simulink model "TestCase_TestSpace_TestSpace_mapping"  (R2016b)
settings: Solver=FixedStepAuto  StartTime=0.0  StopTime=10.0  RelTol=1e-3
model workspace: external: MAT-File TestCase_TestSpace_TestSpace_mapping.mat (data not in the file)
libraries: libTLAsserts x4, libAsserts x2
settings Model: Creator=NEATdemo  LastModifiedBy=NEATdemo

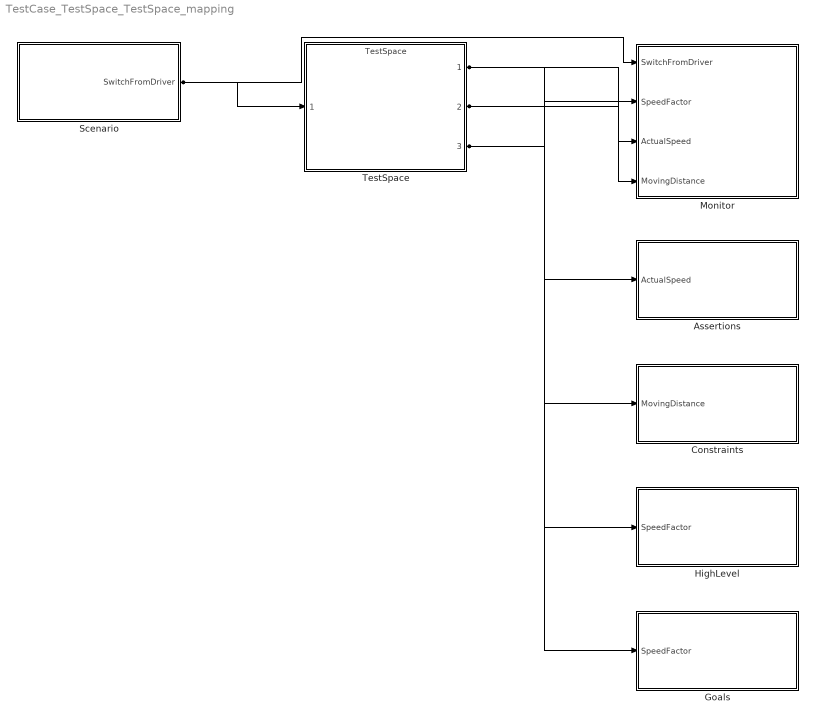
== system TestCase_TestSpace_TestSpace_mapping ==
  Assertions : Subsystem
  Constraints : Subsystem
  Goals : Subsystem
  HighLevel : Subsystem
  Monitor : Subsystem
  Scenario : Subsystem
  TestSpace : ModelReference  ModelNameDialog=TestSpace  SimulationMode=Normal  ModelReferenceVersion=1.13
  wires:
  Scenario/1(SwitchFromDriver) -> TestSpace/1, Monitor/1(SwitchFromDriver)
  TestSpace/3 -> Monitor/2(SpeedFactor), HighLevel/1(SpeedFactor), Goals/1(SpeedFactor)
  TestSpace/2 -> Monitor/3(ActualSpeed), Assertions/1(ActualSpeed)
  TestSpace/1 -> Monitor/4(MovingDistance), Constraints/1(MovingDistance)

== system TestCase_TestSpace_TestSpace_mapping/Assertions ==
  ActualSpeed : Inport
  assert_1 : Subsystem
  simout_1 : ToFile  Filename=assert_1.mat  MatrixName=assert_1  SaveFormat=Timeseries
  wires:
  ActualSpeed/1 -> assert_1/1(ActualSpeed)
  assert_1/1(assert_1_FAILED) -> simout_1/1

== system TestCase_TestSpace_TestSpace_mapping/Constraints ==
  MovingDistance : Inport
  const_1 : Subsystem
  simout_1 : ToFile  Filename=const_1.mat  MatrixName=const_1  SaveFormat=Timeseries
  wires:
  MovingDistance/1 -> const_1/1(MovingDistance)
  const_1/1(const_1_FAILED) -> simout_1/1

== system TestCase_TestSpace_TestSpace_mapping/Goals ==
  SpeedFactor : Inport
  goals_1 : Subsystem
  simout_1 : ToFile  Filename=goals_1.mat  MatrixName=goals_1  SaveFormat=Timeseries
  wires:
  SpeedFactor/1 -> goals_1/1(SpeedFactor)
  goals_1/1(goals_1_VAL) -> simout_1/1

== system TestCase_TestSpace_TestSpace_mapping/HighLevel ==
  SpeedFactor : Inport
  highlevel_1 : Subsystem
  simout_1 : ToFile  Filename=highlevel_1.mat  MatrixName=highlevel_1  SaveFormat=Timeseries
  wires:
  SpeedFactor/1 -> highlevel_1/1(SpeedFactor)
  highlevel_1/1(highlevel_1_FAILED) -> simout_1/1

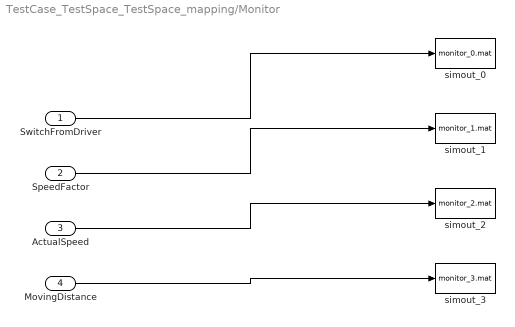
== system TestCase_TestSpace_TestSpace_mapping/Monitor ==
  SwitchFromDriver : Inport
  SpeedFactor : Inport  Port=2
  ActualSpeed : Inport  Port=3
  MovingDistance : Inport  Port=4
  simout_0 : ToFile  Filename=monitor_0.mat  MatrixName=SwitchFromDriver  SaveFormat=Timeseries
  simout_1 : ToFile  Filename=monitor_1.mat  MatrixName=SpeedFactor  SaveFormat=Timeseries
  simout_2 : ToFile  Filename=monitor_2.mat  MatrixName=ActualSpeed  SaveFormat=Timeseries
  simout_3 : ToFile  Filename=monitor_3.mat  MatrixName=MovingDistance  SaveFormat=Timeseries
  wires:
  SwitchFromDriver/1 -> simout_0/1
  SpeedFactor/1 -> simout_1/1
  ActualSpeed/1 -> simout_2/1
  MovingDistance/1 -> simout_3/1

== system TestCase_TestSpace_TestSpace_mapping/Scenario ==
  Scenario : Stateflow chart  TreatAsAtomicUnit=on
  clock : Clock
  SwitchFromDriver : Outport
  wires:
  Scenario/1(SwitchFromDriver) -> SwitchFromDriver/1
  clock/1 -> Scenario/1(clk)

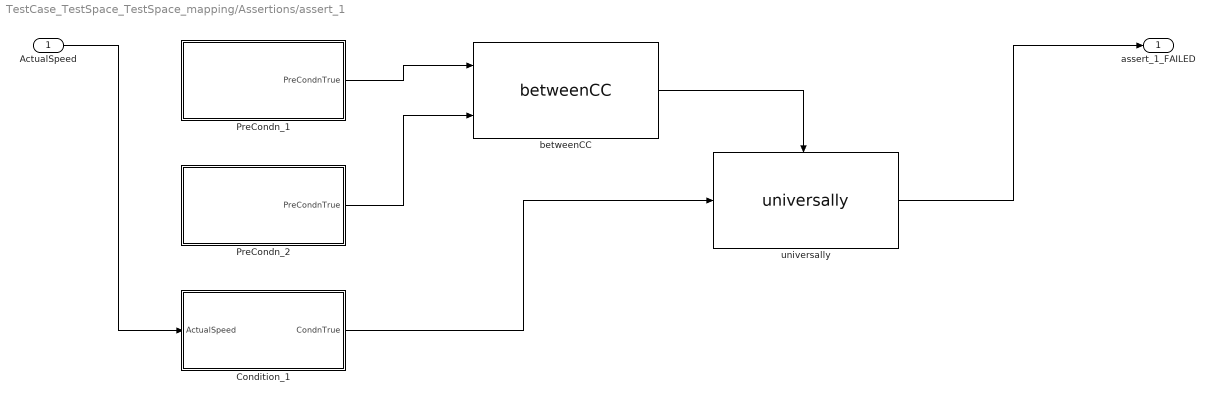
== system TestCase_TestSpace_TestSpace_mapping/Assertions/assert_1 ==
  ActualSpeed : Inport
  Condition_1 : Subsystem
  PreCondn_1 : Subsystem
  PreCondn_2 : Subsystem
  betweenCC : libTLAsserts/betweenCC
  universally : libTLAsserts/universally
  assert_1_FAILED : Outport
  wires:
  ActualSpeed/1 -> Condition_1/1(ActualSpeed)
  PreCondn_1/1(PreCondnTrue) -> betweenCC/1
  PreCondn_2/1(PreCondnTrue) -> betweenCC/2
  Condition_1/1(CondnTrue) -> universally/1
  betweenCC/1 -> universally/Enable
  universally/1 -> assert_1_FAILED/1

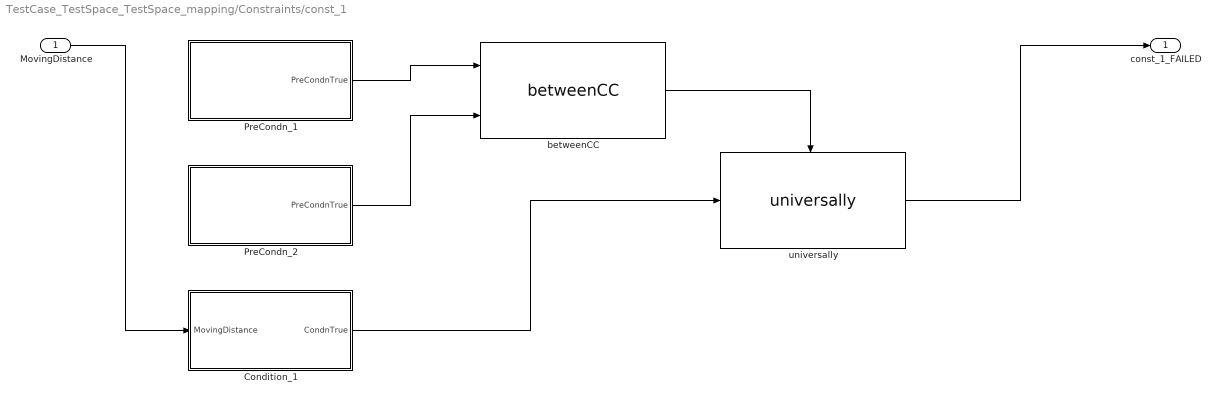
== system TestCase_TestSpace_TestSpace_mapping/Constraints/const_1 ==
  MovingDistance : Inport
  Condition_1 : Subsystem
  PreCondn_1 : Subsystem
  PreCondn_2 : Subsystem
  betweenCC : libTLAsserts/betweenCC
  universally : libTLAsserts/universally
  const_1_FAILED : Outport
  wires:
  MovingDistance/1 -> Condition_1/1(MovingDistance)
  PreCondn_1/1(PreCondnTrue) -> betweenCC/1
  PreCondn_2/1(PreCondnTrue) -> betweenCC/2
  Condition_1/1(CondnTrue) -> universally/1
  betweenCC/1 -> universally/Enable
  universally/1 -> const_1_FAILED/1

== system TestCase_TestSpace_TestSpace_mapping/Goals/goals_1 ==
  SpeedFactor : Inport
  goals_1_VAL : Outport
  wires:
  SpeedFactor/1 -> goals_1_VAL/1

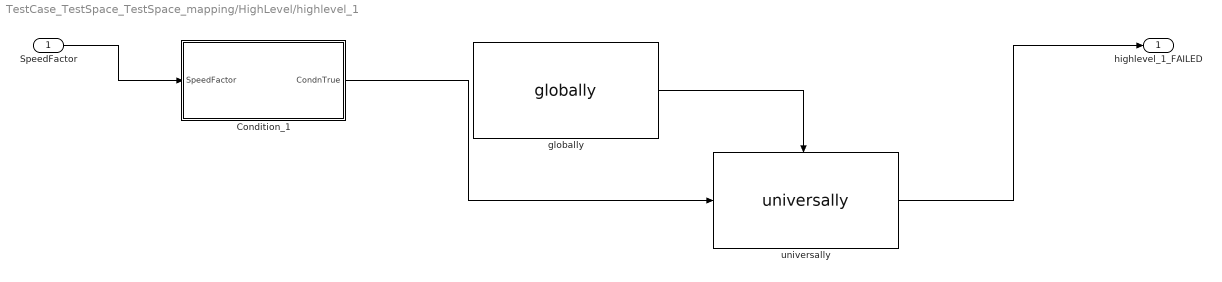
== system TestCase_TestSpace_TestSpace_mapping/HighLevel/highlevel_1 ==
  SpeedFactor : Inport
  Condition_1 : Subsystem
  globally : libAsserts/globally
  universally : libAsserts/universally
  highlevel_1_FAILED : Outport
  wires:
  SpeedFactor/1 -> Condition_1/1(SpeedFactor)
  Condition_1/1(CondnTrue) -> universally/1
  universally/1 -> highlevel_1_FAILED/1
  globally/1 -> universally/Enable

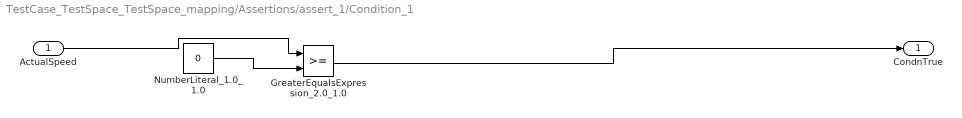
== system TestCase_TestSpace_TestSpace_mapping/Assertions/assert_1/Condition_1 ==
  ActualSpeed : Inport
  GreaterEqualsExpression_2.0_1.0 : RelationalOperator  OutDataTypeStr=boolean  RndMeth=Simplest
  NumberLiteral_1.0_1.0 : Constant  Value=0
  CondnTrue : Outport
  wires:
  ActualSpeed/1 -> GreaterEqualsExpression_2.0_1.0/1
  NumberLiteral_1.0_1.0/1 -> GreaterEqualsExpression_2.0_1.0/2
  GreaterEqualsExpression_2.0_1.0/1 -> CondnTrue/1

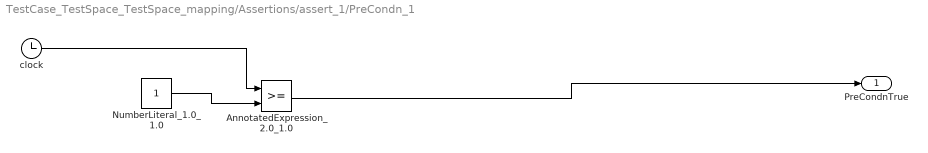
== system TestCase_TestSpace_TestSpace_mapping/Assertions/assert_1/PreCondn_1 ==
  AnnotatedExpression_2.0_1.0 : RelationalOperator  OutDataTypeStr=boolean  RndMeth=Simplest
  NumberLiteral_1.0_1.0 : Constant
  clock : Clock
  PreCondnTrue : Outport
  wires:
  clock/1 -> AnnotatedExpression_2.0_1.0/1
  NumberLiteral_1.0_1.0/1 -> AnnotatedExpression_2.0_1.0/2
  AnnotatedExpression_2.0_1.0/1 -> PreCondnTrue/1

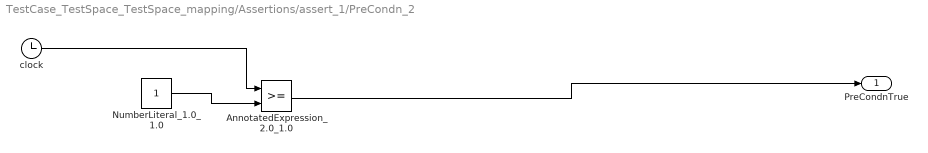
== system TestCase_TestSpace_TestSpace_mapping/Assertions/assert_1/PreCondn_2 ==
  AnnotatedExpression_2.0_1.0 : RelationalOperator  OutDataTypeStr=boolean  RndMeth=Simplest
  NumberLiteral_1.0_1.0 : Constant
  clock : Clock
  PreCondnTrue : Outport
  wires:
  clock/1 -> AnnotatedExpression_2.0_1.0/1
  NumberLiteral_1.0_1.0/1 -> AnnotatedExpression_2.0_1.0/2
  AnnotatedExpression_2.0_1.0/1 -> PreCondnTrue/1

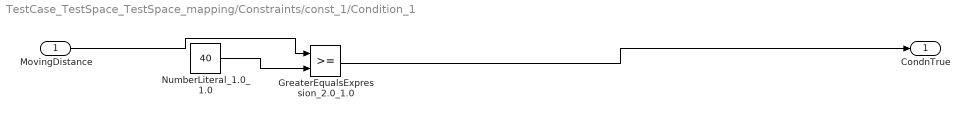
== system TestCase_TestSpace_TestSpace_mapping/Constraints/const_1/Condition_1 ==
  MovingDistance : Inport
  GreaterEqualsExpression_2.0_1.0 : RelationalOperator  OutDataTypeStr=boolean  RndMeth=Simplest
  NumberLiteral_1.0_1.0 : Constant  Value=40
  CondnTrue : Outport
  wires:
  MovingDistance/1 -> GreaterEqualsExpression_2.0_1.0/1
  NumberLiteral_1.0_1.0/1 -> GreaterEqualsExpression_2.0_1.0/2
  GreaterEqualsExpression_2.0_1.0/1 -> CondnTrue/1

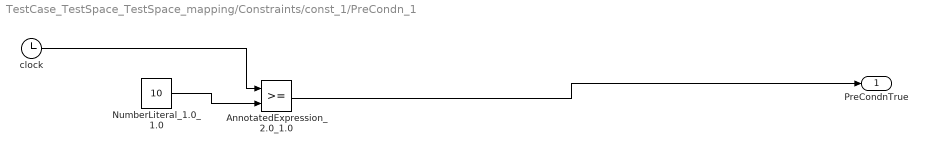
== system TestCase_TestSpace_TestSpace_mapping/Constraints/const_1/PreCondn_1 ==
  AnnotatedExpression_2.0_1.0 : RelationalOperator  OutDataTypeStr=boolean  RndMeth=Simplest
  NumberLiteral_1.0_1.0 : Constant  Value=10
  clock : Clock
  PreCondnTrue : Outport
  wires:
  clock/1 -> AnnotatedExpression_2.0_1.0/1
  NumberLiteral_1.0_1.0/1 -> AnnotatedExpression_2.0_1.0/2
  AnnotatedExpression_2.0_1.0/1 -> PreCondnTrue/1

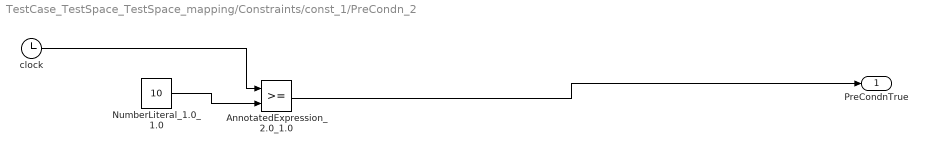
== system TestCase_TestSpace_TestSpace_mapping/Constraints/const_1/PreCondn_2 ==
  AnnotatedExpression_2.0_1.0 : RelationalOperator  OutDataTypeStr=boolean  RndMeth=Simplest
  NumberLiteral_1.0_1.0 : Constant  Value=10
  clock : Clock
  PreCondnTrue : Outport
  wires:
  clock/1 -> AnnotatedExpression_2.0_1.0/1
  NumberLiteral_1.0_1.0/1 -> AnnotatedExpression_2.0_1.0/2
  AnnotatedExpression_2.0_1.0/1 -> PreCondnTrue/1

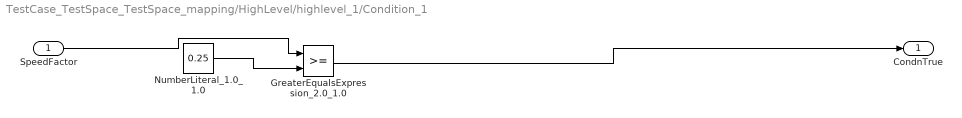
== system TestCase_TestSpace_TestSpace_mapping/HighLevel/highlevel_1/Condition_1 ==
  SpeedFactor : Inport
  GreaterEqualsExpression_2.0_1.0 : RelationalOperator  OutDataTypeStr=boolean  RndMeth=Simplest
  NumberLiteral_1.0_1.0 : Constant  Value=0.25
  CondnTrue : Outport
  wires:
  SpeedFactor/1 -> GreaterEqualsExpression_2.0_1.0/1
  NumberLiteral_1.0_1.0/1 -> GreaterEqualsExpression_2.0_1.0/2
  GreaterEqualsExpression_2.0_1.0/1 -> CondnTrue/1

== stateflow chart TestCase_TestSpace_TestSpace_mapping/Scenario/Scenario ==
  state Act_Controller [parallel]
    settings: executionOrder=1
    state Act_Controller_Step1
    state Act_Controller_Step2
      entry: SwitchFromDriver = 1;
    state Act_Controller_Step3
    (default) -> Act_Controller_Step1
    Act_Controller_Step1 -> Act_Controller_Step2 : [clk >= 1]
    Act_Controller_Step2 -> Act_Controller_Step3
  state Act_Car [parallel]
    settings: executionOrder=2
    state Act_Car_Step1
    (default) -> Act_Car_Step1
  data: clk input; SwitchFromDriver output
